simulink model "pendulum_sim"  (R2015a)
settings: Solver=ode45  StartTime=0.0  StopTime=300  RelTol=1e-3
InitFcn:
  | param
undefined symbols (not defined in the file or in its folder): drawPendulum, P, pendulum_ctrl
settings Model: Creator=beard  LastModifiedBy=beard
settings DataIOCC: SignalLoggingSaveFormat=ModelDataLogs
settings OptimizationCC: ExpressionDepthLimit=2147483647  InitFltsAndDblsToZero=on
settings DebuggingCC: UnderspecifiedInitializationDetection=Classic  MergeDetectMultiDrivingBlocksExec=none  SolverPrmCheckMsg=warning  FcnCallInpInsideContextMsg=UseLocalSettings  StateNameClashWarn=warning
settings GRTTargetCC: CombineOutputUpdateFcns=off  GRTInterface=on

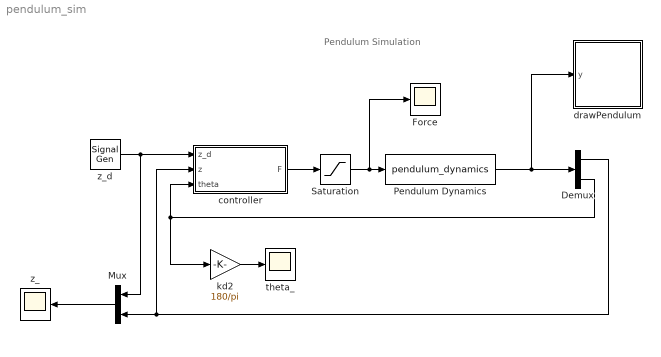
== system pendulum_sim ==
  note: Pendulum Simulation
  Demux : Demux  Outputs=2
  Force : Scope
      settings: TimeRange=49.99  SaveName=ScopeData2
  Mux : Mux  Inputs=2
  Pendulum Dynamics : S-Function  FunctionName=pendulum_dynamics  Parameters=AP
  Saturation : Saturate  UpperLimit=P.F_max  LowerLimit=-P.F_max
  controller : Subsystem
  drawPendulum : Subsystem
      mask Display: image(imread('tv.jpg'))
  kd2 : Gain  Gain=180/pi
  theta_ : Scope
      settings: TimeRange=49.99  YMin=-4  YMax=4
  z_ : Scope
      settings: TimeRange=49.99  YMin=-0.6000000000000001  YMax=0.6000000000000001
  z_d : SignalGenerator  WaveForm=square  Amplitude=0.5  Frequency=.02
  wires:
  Pendulum Dynamics/1 -> Demux/1, drawPendulum/1(y)
  controller/1(F) -> Saturation/1
  Saturation/1 -> Force/1, Pendulum Dynamics/1
  Demux/2 -> controller/3(theta), kd2/1
  Demux/1 -> Mux/2, controller/2(z)
  z_d/1 -> Mux/1, controller/1(z_d)
  Mux/1 -> z_/1
  kd2/1 -> theta_/1

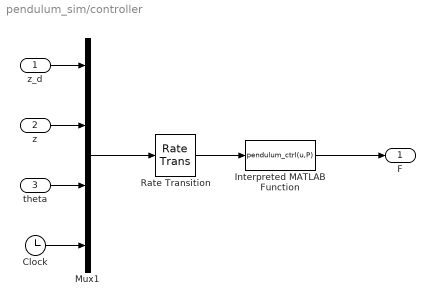
== system pendulum_sim/controller ==
  z_d : Inport
  z : Inport  Port=2
  theta : Inport  Port=3
  Clock : Clock
  Interpreted MATLAB Function : MATLABFcn  MATLABFcn=pendulum_ctrl(u,P)  OutputDimensions=1
  Mux1 : Mux
  Rate Transition : RateTransition  OutPortSampleTime=P.Ts
  F : Outport
  wires:
  Mux1/1 -> Rate Transition/1
  z_d/1 -> Mux1/1
  Interpreted MATLAB Function/1 -> F/1
  Clock/1 -> Mux1/4
  Rate Transition/1 -> Interpreted MATLAB Function/1
  theta/1 -> Mux1/3
  z/1 -> Mux1/2

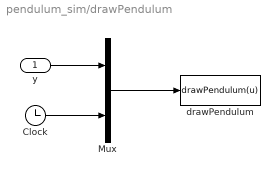
== system pendulum_sim/drawPendulum ==
  y : Inport
  Clock : Clock
  Mux : Mux  Inputs=2
  drawPendulum : MATLABFcn  MATLABFcn=drawPendulum(u)  OutputDimensions=0  SampleTime=0.1
  wires:
  Mux/1 -> drawPendulum/1
  y/1 -> Mux/1
  Clock/1 -> Mux/2
